simulink library "flexy2_lib"  (R2019b)
settings: Solver=VariableStepAuto  StartTime=0.0  StopTime=10.0  RelTol=1e-3
settings Model: Creator=MK  LastModifiedBy=MK
settings DataIOCC: ReturnWorkspaceOutputs=off
settings DebuggingCC: ArithmeticOperatorsInVariantConditions=warning
settings SFSimCC: SimUseLocalCustomCode=off  CustomCodeUndefinedFunction=UseInterfaceOnly
settings RTWCC: RTWUseLocalCustomCode=off

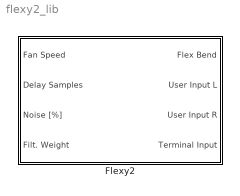
== system flexy2_lib ==
  Flexy2 : Subsystem

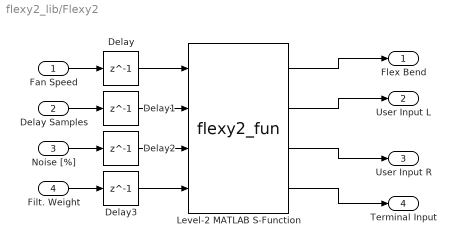
== system flexy2_lib/Flexy2 ==
  Fan Speed : Inport
  Delay Samples : Inport  Port=2
  Noise [%] : Inport  Port=3
  Filt. Weight : Inport  Port=4
  Delay{,1..3} (4 alike) : Delay  DelayLength=1
  Level-2 MATLAB S-Function : M-S-Function  FunctionName=flexy2_fun  Parameters=Ts, Port, calibrate
  Flex Bend : Outport  VectorParamsAs1DForOutWhenUnconnected=off
  User Input L : Outport  Port=2  VectorParamsAs1DForOutWhenUnconnected=off
  User Input R : Outport  Port=3  VectorParamsAs1DForOutWhenUnconnected=off
  Terminal Input : Outport  Port=4  VectorParamsAs1DForOutWhenUnconnected=off
  wires:
  Delay/1 -> Level-2 MATLAB S-Function/1
  Fan Speed/1 -> Delay/1
  Delay Samples/1 -> Delay1/1
  Delay1/1 -> Level-2 MATLAB S-Function/2
  Noise [%]/1 -> Delay2/1
  Delay2/1 -> Level-2 MATLAB S-Function/3
  Level-2 MATLAB S-Function/1 -> Flex Bend/1
  Level-2 MATLAB S-Function/2 -> User Input L/1
  Level-2 MATLAB S-Function/3 -> User Input R/1
  Level-2 MATLAB S-Function/4 -> Terminal Input/1
  Delay3/1 -> Level-2 MATLAB S-Function/4
  Filt. Weight/1 -> Delay3/1
